simulink model "calculator"  (R2017b)
settings: Solver=FixedStepDiscrete  StartTime=0.0  StopTime=10.0  RelTol=1e-3
settings Model: Creator=ebrah  LastModifiedBy=ebrah
settings OptimizationCC: DefaultParameterBehavior=Inlined  PassReuseOutputArgsAs=Individual arguments
settings DebuggingCC: ParameterTunabilityLossMsg=error
settings SFSimCC: MATLABDynamicMemAlloc=off
settings RTWCC: SystemTargetFile=ert.tlc  GenCodeOnly=on  TemplateMakefile=ert_default_tmf  GenerateReport=on  IncludeHyperlinkInReport=on  LaunchReport=on  GenerateTraceInfo=on  GenerateTraceReport=on  GenerateTraceReportSl=on  GenerateTraceReportSf=on  GenerateTraceReportEml=on  GenerateWebview=on
settings CodeAppCC: ForceParamTrailComments=on  IgnoreCustomStorageClasses=off  OperatorAnnotations=on  SimulinkDataObjDesc=on  SFDataObjDesc=on  InsertBlockDesc=on
settings ERTTargetCC: TargetLangStandard=C99 (ISO)  GenerateSampleERTMain=on  InlinedParameterPlacement=NonHierarchical  ERTCustomFileTemplate=example_file_process.tlc

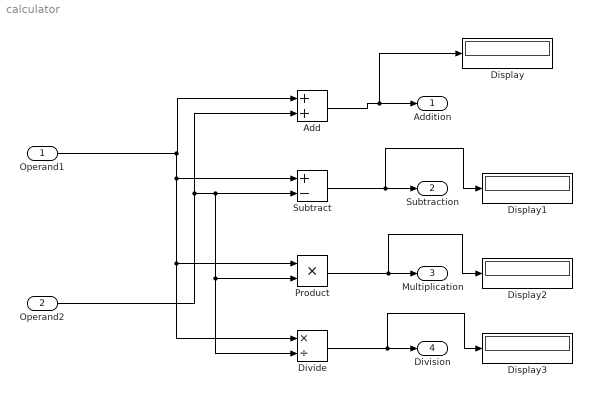
== system calculator ==
  Operand1 : Inport
  Operand2 : Inport  Port=2
  Add : Sum
  Display{,1..3} (4 alike) : Display
  Divide : Product  Inputs=*/
  Product : Product
  Subtract : Sum  Inputs=+-
  Addition : Outport
  Subtraction : Outport  Port=2
  Multiplication : Outport  Port=3
  Division : Outport  Port=4
  wires:
  Operand1/1 -> Divide/1, Product/1, Subtract/1, Add/1
  Operand2/1 -> Divide/2, Product/2, Subtract/2, Add/2
  Add/1 -> Display/1, Addition/1
  Subtract/1 -> Display1/1, Subtraction/1
  Product/1 -> Display2/1, Multiplication/1
  Divide/1 -> Display3/1, Division/1
